simulink model "antenna_OFB_sim_sol"  (R2023b)
settings: Solver=ode3  StartTime=0.0  StopTime=10  FixedStep=0.01  RelTol=1e-3
values from neighbouring files (symbols this model uses):
  A = [ 0 1 ; 0 -a_m ]    [antenna_ADRC_par_sol.m]    (also in antenna_OFB_par_sol.m; pendulum_ADRC_par_sol.m = [ 0 , 1 , 0 ; 0 , 0 , 1 ; 0 , 0 , 0 ])
  B = [ 0 ; Kl*Kg ]    [antenna_ADRC_par_sol.m]    (also in antenna_OFB_par_sol.m; pendulum_ADRC_par_sol.m = [ 0; b0 ; 0 ])
  C = [ 1 , 0 ]    [antenna_ADRC_par_sol.m]    (also in antenna_OFB_par_sol.m; pendulum_ADRC_par_sol.m = [ 1 , 0 , 0 ])
  K = acker(A_cont,B_cont,p_cont)    [antenna_ADRC_par_sol.m]    (also in antenna_OFB_par_sol.m = acker(A,B,p_cont))
  L = acker(A',C',p_obs)'    [antenna_OFB_par_sol.m]    (also in pendulum_ADRC_par_sol.m = acker(A',C',poles_ESO)')
  N_bar = N_u + K*N_x    [antenna_OFB_par_sol.m]
libraries: simulink_extras x3
settings Model: Creator=jerome  LastModifiedBy=jerome
settings ModelReferenceCC: EnableRefExpFcnMdlSchedulingChecks=on

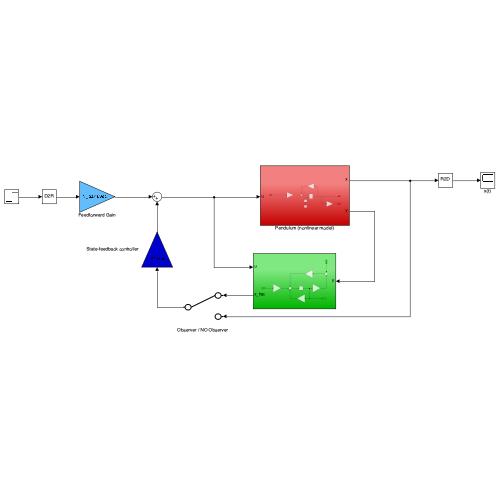
[thumbnail: Simulink's stored preview of the top-level diagram]
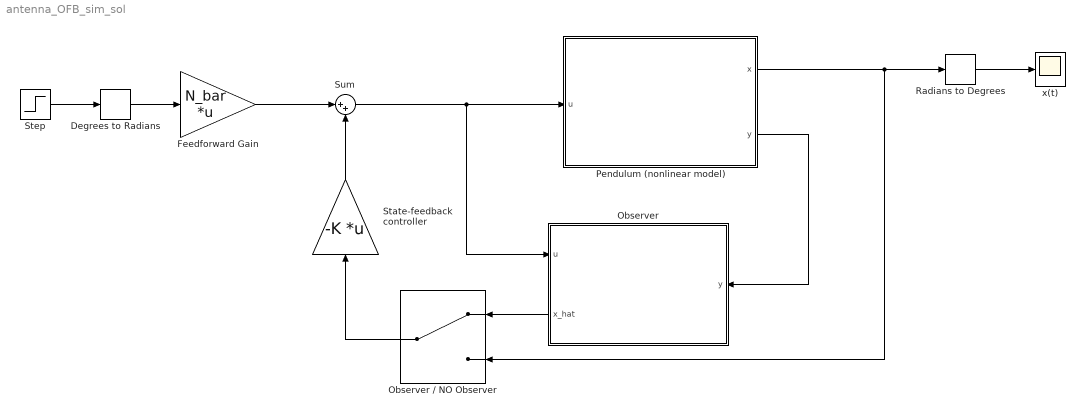
== system antenna_OFB_sim_sol ==
  Degrees to Radians : simulink_extras/Transformations/Degrees to Radians
  Feedforward Gain : Gain  Gain=N_bar  Multiplication=Matrix(K*u) (u vector)
  Observer : Subsystem
      settings: PortSchema="{\"entries\":[{\"content\":{\"sides\":[{\"content\":{\"connectorIds\":[\"In1\",\"Out1\"]},\"type\":\"ConnectorPlacement.EquallySpacedRectSide\",\"uuid\":\"e39c489f-7ce3-4515-bfb3-5978cf16689b\"},{\"content\":{\"connectorIds\":[\"In2\"],\"side\":\"RIGHT\"},\"type\":\"ConnectorPlacement.EquallySpacedRectSide\",\"uuid\":\"c323375b-3042-4327-9d10-0e78d49b9c28\"},{\"content\":{\"connectorIds\":[],\"side\":\"TOP\"},\"type\":\"ConnectorPlacement.EquallySpacedRectSide\",\"uuid\":\"bc6e3c93-589b-408b-8e2a-2332a4933e23\"},{\"content\":{\"connectorIds\":[],\"side\":\"BOTTOM\"},\"type\":\"ConnectorPlacement.EquallySpacedRectSide\",\"uuid\":\"0fa3e6d2-737b-4634-8e4c-4849dc2892cb\"}]},\"type\":\"ConnectorPlacement.EquallySpacedConnector\",\"uuid\":\"052b3b38-b01c-47b0-92b2-1f2c82c768d4\"}],\"packageUris\":[\"http://schema.mathworks.com/mf0/Connector/R2020b\"],\"version\":\"1.0\"}"
  Observer / NO Observer : ManualSwitch
  Pendulum (nonlinear model) : Subsystem
  Radians to Degrees : simulink_extras/Transformations/Radians to Degrees
  State-feedback controller : Gain  Gain=-K  Multiplication=Matrix(K*u) (u vector)
  Step : Step  After=45  SampleTime=0
  Sum : Sum  Inputs=|++
  x(t) : Scope
  wires:
  Pendulum (nonlinear model)/2(y) -> Observer/2(y)
  Sum/1 -> Observer/1(u), Pendulum (nonlinear model)/1(u)
  Feedforward Gain/1 -> Sum/1
  Step/1 -> Degrees to Radians/1
  State-feedback controller/1 -> Sum/2
  Radians to Degrees/1 -> x(t)/1
  Degrees to Radians/1 -> Feedforward Gain/1
  Observer/1(x_hat) -> Observer / NO Observer/1
  Pendulum (nonlinear model)/1(x) -> Observer / NO Observer/2, Radians to Degrees/1
  Observer / NO Observer/1 -> State-feedback controller/1

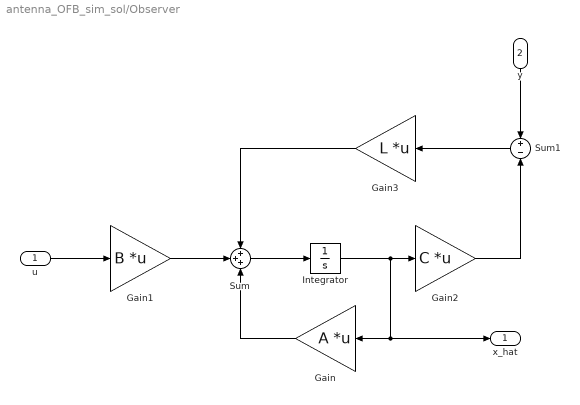
== system antenna_OFB_sim_sol/Observer ==
  u : Inport
  y : Inport  Port=2
  Gain : Gain  Gain=A  Multiplication=Matrix(K*u) (u vector)
  Gain1 : Gain  Gain=B  Multiplication=Matrix(K*u) (u vector)
  Gain2 : Gain  Gain=C  Multiplication=Matrix(K*u) (u vector)
  Gain3 : Gain  Gain=L  Multiplication=Matrix(K*u) (u vector)
  Integrator : Integrator  InitialCondition=zeros(2,1)
  Sum : Sum  Inputs=+++
  Sum1 : Sum  Inputs=+-
  x_hat : Outport
  wires:
  Integrator/1 -> Gain2/1, x_hat/1, Gain/1
  Sum/1 -> Integrator/1
  u/1 -> Gain1/1
  Gain/1 -> Sum/3
  Gain1/1 -> Sum/2
  Gain3/1 -> Sum/1
  Sum1/1 -> Gain3/1
  Gain2/1 -> Sum1/2
  y/1 -> Sum1/1

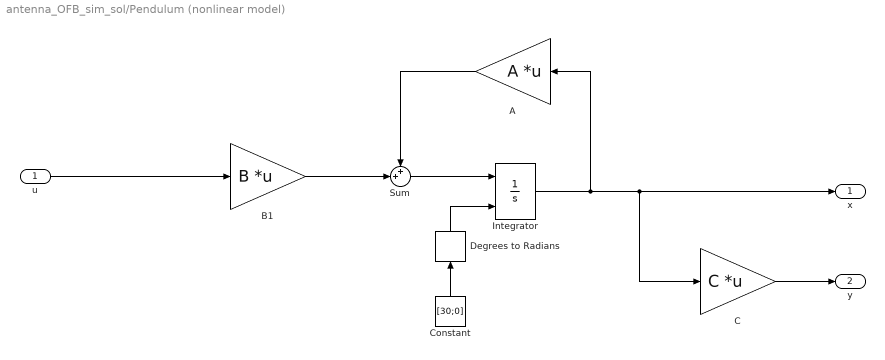
== system antenna_OFB_sim_sol/Pendulum (nonlinear model) ==
  u : Inport
  A : Gain  Gain=A  Multiplication=Matrix(K*u) (u vector)
  B1 : Gain  Gain=B  Multiplication=Matrix(K*u) (u vector)
  C : Gain  Gain=C  Multiplication=Matrix(K*u) (u vector)
  Constant : Constant  Value=[30;0]  VectorParams1D=off
  Degrees to Radians : simulink_extras/Transformations/Degrees to Radians
  Integrator : Integrator  InitialConditionSource=external  InitialCondition=[0.1;0]
  Sum : Sum  Inputs=++|
  x : Outport
  y : Outport  Port=2
  wires:
  Sum/1 -> Integrator/1
  Integrator/1 -> A/1, C/1, x/1
  C/1 -> y/1
  Constant/1 -> Degrees to Radians/1
  Degrees to Radians/1 -> Integrator/2
  A/1 -> Sum/1
  B1/1 -> Sum/2
  u/1 -> B1/1
